simulink model "angle_cnl"  (R2016b)
settings: Solver=VariableStepAuto  StartTime=0.0  StopTime=10.0  RelTol=1e-3
values from neighbouring files (symbols this model uses):
  Acl = A - B*k    [sara.m]
  B = [0;0.2263;0;-0.3565]    [4_5864020115967706803.m]    (also in NYQ.m; Nq_cntrl.m; Nquist.m; main.m)
  k = 1    [4_5864020115967706803.m]    (also in main.m = place(A,B,P); part_2.m; sara.m = place(A,B,P))
  Kf = 1/Kdc    [sara.m]
settings Model: Creator=ASUS  LastModifiedBy=ASUS

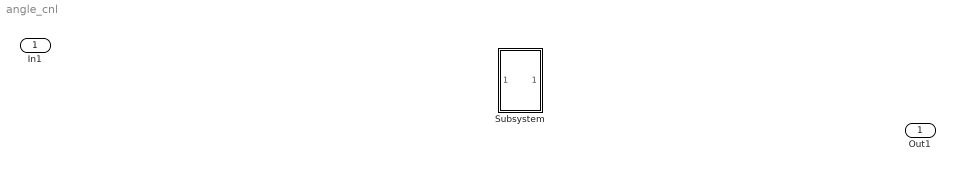
== system angle_cnl ==
  In1 : Inport
  Subsystem : Subsystem
  Out1 : Outport

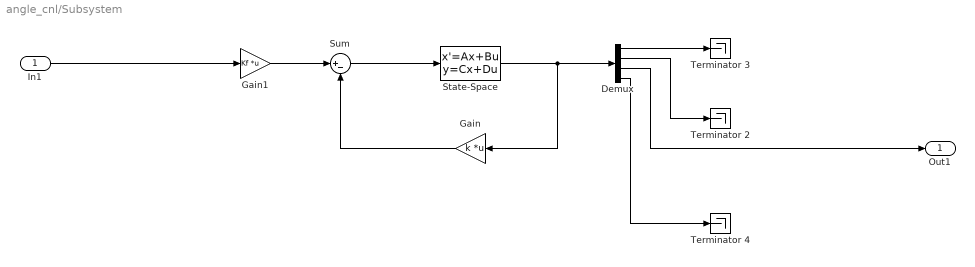
== system angle_cnl/Subsystem ==
  In1 : Inport
  Demux : Demux
  Gain : Gain  Gain=k  Multiplication=Matrix(K*u)
  Gain1 : Gain  Gain=Kf  Multiplication=Matrix(K*u)
  State-Space : StateSpace  A=Acl  B=B  C=eye(4)  D=[0;0;0;0]  X0=0
  Sum : Sum  Inputs=|+-
  Terminator 2 : Terminator
  Terminator 3 : Terminator
  "Terminator 4 " : Terminator
  Out1 : Outport
  wires:
  Demux/1 -> Terminator 3/1
  Demux/2 -> Terminator 2/1
  Demux/4 -> "Terminator 4 "/1
  In1/1 -> Gain1/1
  State-Space/1 -> Gain/1, Demux/1
  Gain1/1 -> Sum/1
  Gain/1 -> Sum/2
  Sum/1 -> State-Space/1
  Demux/3 -> Out1/1
